simulink model "Demo_1_3Q_ST250"  (Simulink 7.7)
settings: Solver=ode4  StartTime=0.0  StopTime=inf  FixedStep=sample_time_Vicon  RelTol=1e-3
InitFcn:
  | sample_time_Vicon = 0.004;
  | sample_time=0.02;
  | DeltaT = sample_time;
  | H0 = -0.36;
  | Kl = 1;
  | Omega_r =1.1; %1.3
undefined symbols (not defined in the file or in its folder): DiscIntNeverNeededParam
libraries: simulink x19, dspadpt3 x8
(part 3 of 3)

== system Demo_1_3Q_ST250/Vicon_Data1/Raw Quad Pose from Vicon/Process Vicon Raw Data3/Flip_pi1/Flip_0_to_2pi ==
  Angle : Inport
  Add : Sum
  Compare To Constant1 : simulink/Logic and Bit Operations/Compare To Constant  SystemSampleTime=-1  relop=<  const=0  LogicOutDataTypeMode=uint8  ZeroCross=off
  Constant : Constant  Value=2*pi
  Data Type Duplicate : DataTypeDuplicate
  Flip_2pi : Subsystem
      mask Type: Flip -2pi to 2pi
      mask Description: Flips the inputs into the range -2pi to +2pi
      mask Help: Flips the inputs into the range -2pi to +2pi
      mask Display: disp('Flip_2pi')
  Switch : Switch  Criteria=u2 ~= 0
  Angle_Flip : Outport
  wires:
  Flip_2pi/1(Angle_Flip) -> Compare To Constant1/1, Add/2, Switch/3
  Compare To Constant1/1 -> Switch/2
  Constant/1 -> Add/1
  Add/1 -> Switch/1
  Angle/1 -> Flip_2pi/1(Angle), Data Type Duplicate/2
  Switch/1 -> Angle_Flip/1, Data Type Duplicate/1

== system Demo_1_3Q_ST250/Vicon_Data1/Raw Quad Pose from Vicon/Process Vicon Raw Data4/Flip_pi1/Flip_0_to_2pi ==
  Angle : Inport
  Add : Sum
  Compare To Constant1 : simulink/Logic and Bit Operations/Compare To Constant  SystemSampleTime=-1  relop=<  const=0  LogicOutDataTypeMode=uint8  ZeroCross=off
  Constant : Constant  Value=2*pi
  Data Type Duplicate : DataTypeDuplicate
  Flip_2pi : Subsystem
      mask Type: Flip -2pi to 2pi
      mask Description: Flips the inputs into the range -2pi to +2pi
      mask Help: Flips the inputs into the range -2pi to +2pi
      mask Display: disp('Flip_2pi')
  Switch : Switch  Criteria=u2 ~= 0
  Angle_Flip : Outport
  wires:
  Switch/1 -> Data Type Duplicate/1, Angle_Flip/1
  Angle/1 -> Data Type Duplicate/2, Flip_2pi/1(Angle)
  Add/1 -> Switch/1
  Constant/1 -> Add/1
  Compare To Constant1/1 -> Switch/2
  Flip_2pi/1(Angle_Flip) -> Switch/3, Add/2, Compare To Constant1/1

== system Demo_1_3Q_ST250/Vicon_Data1/Raw Quad Pose from Vicon/Process Vicon Raw Data5/Flip_pi1/Flip_0_to_2pi ==
  Angle : Inport
  Add : Sum
  Compare To Constant1 : simulink/Logic and Bit Operations/Compare To Constant  SystemSampleTime=-1  relop=<  const=0  LogicOutDataTypeMode=uint8  ZeroCross=off
  Constant : Constant  Value=2*pi
  Data Type Duplicate : DataTypeDuplicate
  Flip_2pi : Subsystem
      mask Type: Flip -2pi to 2pi
      mask Description: Flips the inputs into the range -2pi to +2pi
      mask Help: Flips the inputs into the range -2pi to +2pi
      mask Display: disp('Flip_2pi')
  Switch : Switch  Criteria=u2 ~= 0
  Angle_Flip : Outport
  wires:
  Switch/1 -> Data Type Duplicate/1, Angle_Flip/1
  Angle/1 -> Data Type Duplicate/2, Flip_2pi/1(Angle)
  Add/1 -> Switch/1
  Constant/1 -> Add/1
  Compare To Constant1/1 -> Switch/2
  Flip_2pi/1(Angle_Flip) -> Switch/3, Add/2, Compare To Constant1/1

== system Demo_1_3Q_ST250/Vicon_Data1/Raw Quad Pose from Vicon/Process Vicon Raw Data6/Flip_pi1/Flip_0_to_2pi ==
  Angle : Inport
  Add : Sum
  Compare To Constant1 : simulink/Logic and Bit Operations/Compare To Constant  SystemSampleTime=-1  relop=<  const=0  LogicOutDataTypeMode=uint8  ZeroCross=off
  Constant : Constant  Value=2*pi
  Data Type Duplicate : DataTypeDuplicate
  Flip_2pi : Subsystem
      mask Type: Flip -2pi to 2pi
      mask Description: Flips the inputs into the range -2pi to +2pi
      mask Help: Flips the inputs into the range -2pi to +2pi
      mask Display: disp('Flip_2pi')
  Switch : Switch  Criteria=u2 ~= 0
  Angle_Flip : Outport
  wires:
  Flip_2pi/1(Angle_Flip) -> Compare To Constant1/1, Add/2, Switch/3
  Compare To Constant1/1 -> Switch/2
  Constant/1 -> Add/1
  Add/1 -> Switch/1
  Angle/1 -> Flip_2pi/1(Angle), Data Type Duplicate/2
  Switch/1 -> Angle_Flip/1, Data Type Duplicate/1

== system Demo_1_3Q_ST250/Vicon_Data1/Raw Quad Pose from Vicon/Process Vicon Raw Data7/Flip_pi1/Flip_0_to_2pi ==
  Angle : Inport
  Add : Sum
  Compare To Constant1 : simulink/Logic and Bit Operations/Compare To Constant  SystemSampleTime=-1  relop=<  const=0  LogicOutDataTypeMode=uint8  ZeroCross=off
  Constant : Constant  Value=2*pi
  Data Type Duplicate : DataTypeDuplicate
  Flip_2pi : Subsystem
      mask Type: Flip -2pi to 2pi
      mask Description: Flips the inputs into the range -2pi to +2pi
      mask Help: Flips the inputs into the range -2pi to +2pi
      mask Display: disp('Flip_2pi')
  Switch : Switch  Criteria=u2 ~= 0
  Angle_Flip : Outport
  wires:
  Switch/1 -> Data Type Duplicate/1, Angle_Flip/1
  Angle/1 -> Data Type Duplicate/2, Flip_2pi/1(Angle)
  Add/1 -> Switch/1
  Constant/1 -> Add/1
  Compare To Constant1/1 -> Switch/2
  Flip_2pi/1(Angle_Flip) -> Switch/3, Add/2, Compare To Constant1/1

== system Demo_1_3Q_ST250/Vicon_Data1/Raw Quad Pose from Vicon/Process Vicon Raw Data8/Flip_pi1/Flip_0_to_2pi ==
  Angle : Inport
  Add : Sum
  Compare To Constant1 : simulink/Logic and Bit Operations/Compare To Constant  SystemSampleTime=-1  relop=<  const=0  LogicOutDataTypeMode=uint8  ZeroCross=off
  Constant : Constant  Value=2*pi
  Data Type Duplicate : DataTypeDuplicate
  Flip_2pi : Subsystem
      mask Type: Flip -2pi to 2pi
      mask Description: Flips the inputs into the range -2pi to +2pi
      mask Help: Flips the inputs into the range -2pi to +2pi
      mask Display: disp('Flip_2pi')
  Switch : Switch  Criteria=u2 ~= 0
  Angle_Flip : Outport
  wires:
  Flip_2pi/1(Angle_Flip) -> Compare To Constant1/1, Add/2, Switch/3
  Compare To Constant1/1 -> Switch/2
  Constant/1 -> Add/1
  Add/1 -> Switch/1
  Angle/1 -> Flip_2pi/1(Angle), Data Type Duplicate/2
  Switch/1 -> Angle_Flip/1, Data Type Duplicate/1

== system Demo_1_3Q_ST250/Vicon_Data1/Raw Quad Pose from Vicon/Process Vicon Raw Data1/Flip_pi1/Flip_0_to_2pi/Flip_2pi ==
  Angle : Inport
  Bias : Bias  Bias=-2*pi
  Constant : Constant  Value=2*pi
  Data Type Duplicate : DataTypeDuplicate
  Modulo : Math  Operator=mod  SaturateOnIntegerOverflow=on
  Sign1 : Signum
  Switch : Switch
  Angle_Flip : Outport
  wires:
  Angle/1 -> Modulo/1, Sign1/1, Data Type Duplicate/1
  Constant/1 -> Modulo/2
  Modulo/1 -> Bias/1, Switch/1
  Sign1/1 -> Switch/2
  Bias/1 -> Switch/3
  Switch/1 -> Angle_Flip/1, Data Type Duplicate/2

== system Demo_1_3Q_ST250/Vicon_Data1/Raw Quad Pose from Vicon/Process Vicon Raw Data2/Flip_pi1/Flip_0_to_2pi/Flip_2pi ==
  Angle : Inport
  Bias : Bias  Bias=-2*pi
  Constant : Constant  Value=2*pi
  Data Type Duplicate : DataTypeDuplicate
  Modulo : Math  Operator=mod  SaturateOnIntegerOverflow=on
  Sign1 : Signum
  Switch : Switch
  Angle_Flip : Outport
  wires:
  Switch/1 -> Data Type Duplicate/2, Angle_Flip/1
  Bias/1 -> Switch/3
  Sign1/1 -> Switch/2
  Modulo/1 -> Switch/1, Bias/1
  Constant/1 -> Modulo/2
  Angle/1 -> Data Type Duplicate/1, Sign1/1, Modulo/1

== system Demo_1_3Q_ST250/Vicon_Data1/Raw Quad Pose from Vicon/Process Vicon Raw Data3/Flip_pi1/Flip_0_to_2pi/Flip_2pi ==
  Angle : Inport
  Bias : Bias  Bias=-2*pi
  Constant : Constant  Value=2*pi
  Data Type Duplicate : DataTypeDuplicate
  Modulo : Math  Operator=mod  SaturateOnIntegerOverflow=on
  Sign1 : Signum
  Switch : Switch
  Angle_Flip : Outport
  wires:
  Angle/1 -> Modulo/1, Sign1/1, Data Type Duplicate/1
  Constant/1 -> Modulo/2
  Modulo/1 -> Bias/1, Switch/1
  Sign1/1 -> Switch/2
  Bias/1 -> Switch/3
  Switch/1 -> Angle_Flip/1, Data Type Duplicate/2

== system Demo_1_3Q_ST250/Vicon_Data1/Raw Quad Pose from Vicon/Process Vicon Raw Data4/Flip_pi1/Flip_0_to_2pi/Flip_2pi ==
  Angle : Inport
  Bias : Bias  Bias=-2*pi
  Constant : Constant  Value=2*pi
  Data Type Duplicate : DataTypeDuplicate
  Modulo : Math  Operator=mod  SaturateOnIntegerOverflow=on
  Sign1 : Signum
  Switch : Switch
  Angle_Flip : Outport
  wires:
  Switch/1 -> Data Type Duplicate/2, Angle_Flip/1
  Bias/1 -> Switch/3
  Sign1/1 -> Switch/2
  Modulo/1 -> Switch/1, Bias/1
  Constant/1 -> Modulo/2
  Angle/1 -> Data Type Duplicate/1, Sign1/1, Modulo/1

== system Demo_1_3Q_ST250/Vicon_Data1/Raw Quad Pose from Vicon/Process Vicon Raw Data5/Flip_pi1/Flip_0_to_2pi/Flip_2pi ==
  Angle : Inport
  Bias : Bias  Bias=-2*pi
  Constant : Constant  Value=2*pi
  Data Type Duplicate : DataTypeDuplicate
  Modulo : Math  Operator=mod  SaturateOnIntegerOverflow=on
  Sign1 : Signum
  Switch : Switch
  Angle_Flip : Outport
  wires:
  Switch/1 -> Data Type Duplicate/2, Angle_Flip/1
  Bias/1 -> Switch/3
  Sign1/1 -> Switch/2
  Modulo/1 -> Switch/1, Bias/1
  Constant/1 -> Modulo/2
  Angle/1 -> Data Type Duplicate/1, Sign1/1, Modulo/1

== system Demo_1_3Q_ST250/Vicon_Data1/Raw Quad Pose from Vicon/Process Vicon Raw Data6/Flip_pi1/Flip_0_to_2pi/Flip_2pi ==
  Angle : Inport
  Bias : Bias  Bias=-2*pi
  Constant : Constant  Value=2*pi
  Data Type Duplicate : DataTypeDuplicate
  Modulo : Math  Operator=mod  SaturateOnIntegerOverflow=on
  Sign1 : Signum
  Switch : Switch
  Angle_Flip : Outport
  wires:
  Angle/1 -> Modulo/1, Sign1/1, Data Type Duplicate/1
  Constant/1 -> Modulo/2
  Modulo/1 -> Bias/1, Switch/1
  Sign1/1 -> Switch/2
  Bias/1 -> Switch/3
  Switch/1 -> Angle_Flip/1, Data Type Duplicate/2

== system Demo_1_3Q_ST250/Vicon_Data1/Raw Quad Pose from Vicon/Process Vicon Raw Data7/Flip_pi1/Flip_0_to_2pi/Flip_2pi ==
  Angle : Inport
  Bias : Bias  Bias=-2*pi
  Constant : Constant  Value=2*pi
  Data Type Duplicate : DataTypeDuplicate
  Modulo : Math  Operator=mod  SaturateOnIntegerOverflow=on
  Sign1 : Signum
  Switch : Switch
  Angle_Flip : Outport
  wires:
  Switch/1 -> Data Type Duplicate/2, Angle_Flip/1
  Bias/1 -> Switch/3
  Sign1/1 -> Switch/2
  Modulo/1 -> Switch/1, Bias/1
  Constant/1 -> Modulo/2
  Angle/1 -> Data Type Duplicate/1, Sign1/1, Modulo/1

== system Demo_1_3Q_ST250/Vicon_Data1/Raw Quad Pose from Vicon/Process Vicon Raw Data8/Flip_pi1/Flip_0_to_2pi/Flip_2pi ==
  Angle : Inport
  Bias : Bias  Bias=-2*pi
  Constant : Constant  Value=2*pi
  Data Type Duplicate : DataTypeDuplicate
  Modulo : Math  Operator=mod  SaturateOnIntegerOverflow=on
  Sign1 : Signum
  Switch : Switch
  Angle_Flip : Outport
  wires:
  Angle/1 -> Modulo/1, Sign1/1, Data Type Duplicate/1
  Constant/1 -> Modulo/2
  Modulo/1 -> Bias/1, Switch/1
  Sign1/1 -> Switch/2
  Bias/1 -> Switch/3
  Switch/1 -> Angle_Flip/1, Data Type Duplicate/2

== matlab function Quad 1 Planning/Yaw Controller/MATLAB Function ==
  data: u input double; y output double
function y = fcn(u)
%#codegen
y = u;
if y > pi    
    y = y - 2*pi;
elseif y < -pi
        y = y + 2*pi;
end

== stateflow chart Quad 2 Planning/Trajectory Logic/UAV SF ==
  state Landing
    state Decsending
      en:PosDesired = Pos;
      du:PosDesired[2] = (0 - PosDesired[2])*1*DeltaT + PosDesired[2] ;
    state CutThrottle
      du:HoverThrottle = (-0.95 - HoverThrottle)*2*DeltaT + HoverThrottle ;
    (default) -> Decsending
    Decsending -> CutThrottle : [Pos[2] > -0.15]
  state Airborne
    state TakeOff
      du:HoverThrottle = (H0 - HoverThrottle)*2*DeltaT + HoverThrottle ;
    state Hover
      en: PosDesired[2] = -1;
    state Line
      state Waypoint2
        en: PosDesired[0] = 0; PosDesired[1] = -1.7321-0.5;  PosDesired[2] = -2;
      state Waypoint1
        en: PosDesired[0] = 0; PosDesired[1] = 1.7321-0.5; PosDesired[2] = -1;
        line_count = line_count+1;
      (default) -> Airborne.Line.Waypoint1 : {line_count = -1;}
      Airborne.Line.Waypoint2 -> Airborne.Line.Waypoint1 : after(5,sec)
      Airborne.Line.Waypoint1 -> Airborne.Line.Waypoint2 : after(5,sec)
    state Triangle_CW
      state Waypoint3
        en:PosDesired[0] = -2;
        PosDesired[1] = 1.7321-0.5;
        PosDesired[2] = -1;
      state Waypoint2
        en:PosDesired[0] = 2;
        PosDesired[1] = 1.7321-0.5;
        PosDesired[2] = -1.5;
        triangle_count = triangle_count + 1;
      state Waypoint1
        en:PosDesired[0] = 0;
        PosDesired[1] = -1.7321-0.5;
        PosDesired[2] = -2.0;
      (default) -> Airborne.Triangle_CW.Waypoint2 : {triangle_count = -1;}
      Airborne.Triangle_CW.Waypoint3 -> Airborne.Triangle_CW.Waypoint1 : after(5,sec)
      Airborne.Triangle_CW.Waypoint2 -> Airborne.Triangle_CW.Waypoint3 : after(5,sec)
      Airborne.Triangle_CW.Waypoint1 -> Airborne.Triangle_CW.Waypoint2 : after(5,sec)
    state Triangle_CCW
      state Waypoint3
        en:PosDesired[0] = 2;
        PosDesired[1] = 1.7321-0.5;
        PosDesired[2] = -1.5;
      state Waypoint1
        en:PosDesired[0] = 0;
        PosDesired[1] = -1.7321-0.5;
        PosDesired[2] = -2.0;
      state Waypoint2
        en:PosDesired[0] = -2;
        PosDesired[1] = 1.7321-0.5;
        PosDesired[2] = -1;
        triangle_count = triangle_count + 1;
      Airborne.Triangle_CCW.Waypoint3 -> Airborne.Triangle_CCW.Waypoint1 : after(5,sec)
      (default) -> Airborne.Triangle_CCW.Waypoint1 : {triangle_count = -1;}
      Airborne.Triangle_CCW.Waypoint2 -> Airborne.Triangle_CCW.Waypoint3 : after(5,sec)
      Airborne.Triangle_CCW.Waypoint1 -> Airborne.Triangle_CCW.Waypoint2 : after(5,sec)
    (default) -> TakeOff : {PosDesired = Pos;  PosDesired[2] = -1;}
    TakeOff -> Hover : after(5,sec)
        | {PosDesired = Pos;}
    Hover -> Line : [RC[5] > 0]
    Triangle_CW -> Hover [order 2] : [RC[5] < 0]
        | {PosDesired = Pos;}
    Line -> Triangle_CCW [order 1] : [line_count == 2]
    Line -> Hover [order 2] : [RC[5] < 0]
        | {PosDesired = Pos;}
    Triangle_CW -> Hover [order 1] : [triangle_count == 2]
    Triangle_CCW -> Hover [order 1] : [RC[5] < 0]
        | {PosDesired = Pos;}
    Triangle_CCW -> Triangle_CW [order 2] : [triangle_count == 2]
  (default) -> Landing : {HoverThrottle=-0.95;}
  Airborne -> Landing : [RC[6] < -0.5]
  Landing -> Airborne : [RC[6] > 0.5]
  data: PosDesired output double size=4; HoverThrottle output double size=1; Mode output uint8 size=3; RC input double size=8; Pos input double size=4; PerchPos input double size=4; DeltaT parameter double size=1; H0 parameter double size=1; Kl parameter double size=1; VelCmd local double size=2 =0; line_count local int8 size=1 =0; triangle_count local int8 size=1 =0

== stateflow chart Quad 1 Planning/Trajectory Logic/UAV SF ==
  state Landing
    state Decsending
      en:PosDesired = Pos;
      du:PosDesired[2] = (0 - PosDesired[2])*1*DeltaT + PosDesired[2] ;
    state CutThrottle
      du:HoverThrottle = (-0.95 - HoverThrottle)*2*DeltaT + HoverThrottle ;
    (default) -> Decsending
    Decsending -> CutThrottle : [Pos[2] > -0.15]
  state Airborne
    state TakeOff
      du:HoverThrottle = (H0 - HoverThrottle)*2*DeltaT + HoverThrottle ;
    state Hover
      en: PosDesired[2] = -1;
    state Line
      state Waypoint2
        en: PosDesired[0] = 2; PosDesired[1] = -1.7321-0.5;  PosDesired[2] = -2;
      state Waypoint1
        en: PosDesired[0] = 2; PosDesired[1] = 1.7321-0.5; PosDesired[2] = -1;
        line_count = line_count+1;
      (default) -> Airborne.Line.Waypoint1 : {line_count = -1;}
      Airborne.Line.Waypoint2 -> Airborne.Line.Waypoint1 : after(5,sec)
      Airborne.Line.Waypoint1 -> Airborne.Line.Waypoint2 : after(5,sec)
    state Triangle_CW
      state Waypoint2
        en:PosDesired[0] = -2;
        PosDesired[1] = 1.7321-0.5;
        PosDesired[2] = -1;
        triangle_count = triangle_count + 1;
      state Waypoint1
        en:PosDesired[0] = 2;
        PosDesired[1] = 1.7321-0.5;
        PosDesired[2] = -1.5;
      state Waypoint3
        en:PosDesired[0] = 0;
        PosDesired[1] = -1.7321-0.5;
        PosDesired[2] = -2.0;
      (default) -> Airborne.Triangle_CW.Waypoint2 : {triangle_count = -1;}
      Airborne.Triangle_CW.Waypoint1 -> Airborne.Triangle_CW.Waypoint2 : after(5,sec)
      Airborne.Triangle_CW.Waypoint2 -> Airborne.Triangle_CW.Waypoint3 : after(5,sec)
      Airborne.Triangle_CW.Waypoint3 -> Airborne.Triangle_CW.Waypoint1 : after(5,sec)
    state Triangle_CCW
      state Waypoint3
        en:PosDesired[0] = -2;
        PosDesired[1] = 1.7321-0.5;
        PosDesired[2] = -1;
      state Waypoint1
        en:PosDesired[0] = 2;
        PosDesired[1] = 1.7321-0.5;
        PosDesired[2] = -1.5;
      state Waypoint2
        en:PosDesired[0] = 0;
        PosDesired[1] = -1.7321-0.5;
        PosDesired[2] = -2.0;
        triangle_count = triangle_count + 1;
      Airborne.Triangle_CCW.Waypoint1 -> Airborne.Triangle_CCW.Waypoint2 : after(5,sec)
      Airborne.Triangle_CCW.Waypoint3 -> Airborne.Triangle_CCW.Waypoint1 : after(5,sec)
      (default) -> Airborne.Triangle_CCW.Waypoint1 : {triangle_count = -1;}
      Airborne.Triangle_CCW.Waypoint2 -> Airborne.Triangle_CCW.Waypoint3 : after(5,sec)
    (default) -> TakeOff : {PosDesired = Pos;  PosDesired[2] = -1;}
    TakeOff -> Hover : after(5,sec)
        | {PosDesired = Pos;}
    Hover -> Line : [RC[5] > 0]
    Triangle_CW -> Hover [order 2] : [RC[5] < 0]
        | {PosDesired = Pos;}
    Triangle_CCW -> Triangle_CW [order 2] : [triangle_count == 2]
    Triangle_CCW -> Hover [order 1] : [RC[5] < 0]
        | {PosDesired = Pos;}
    Line -> Triangle_CCW [order 1] : [line_count == 2]
    Line -> Hover [order 2] : [RC[5] < 0]
        | {PosDesired = Pos;}
    Triangle_CW -> Hover [order 1] : [triangle_count == 2]
  (default) -> Landing : {HoverThrottle=-0.95;}
  Airborne -> Landing : [RC[6] < -0.5]
  Landing -> Airborne : [RC[6] > 0.5]
  data: PosDesired output double size=4; HoverThrottle output double size=1; Mode output uint8 size=3; RC input double size=8; Pos input double size=4; PerchPos input double size=4; DeltaT parameter double size=1; H0 parameter double size=1; Kl parameter double size=1; VelCmd local double size=2 =0; line_count local int8 size=1 =0; triangle_count local int8 size=1 =0

== matlab function Quad 2 Planning/Yaw Controller/MATLAB Function ==
  data: u input double; y output double
function y = fcn(u)
%#codegen
y = u;
if y > pi    
    y = y - 2*pi;
elseif y < -pi
        y = y + 2*pi;
end

== stateflow chart Quad 4 Planning (same as Q3)/Trajectory Logic/UAV SF ==
  state Landing
    state Decsending
      en:PosDesired = Pos;
      du:PosDesired[2] = (0 - PosDesired[2])*1*DeltaT + PosDesired[2] ;
    state CutThrottle
      du:HoverThrottle = (-0.95 - HoverThrottle)*2*DeltaT + HoverThrottle ;
    (default) -> Decsending
    Decsending -> CutThrottle : [Pos[2] > -0.15]
  state Airborne
    state TakeOff
      du:HoverThrottle = (-0.27 - HoverThrottle)*2*DeltaT + HoverThrottle ;
    state Hover
      en: PosDesired[2] = -1;
    state Line
      state Waypoint2
        en: PosDesired[0] = -2; PosDesired[1] = -1.7321-0.5;  PosDesired[2] = -2;
      state Waypoint1
        en: PosDesired[0] = -2; PosDesired[1] = 1.7321-0.5; PosDesired[2] = -1;
        line_count = line_count+1;
      (default) -> Airborne.Line.Waypoint1 : {line_count = -1;}
      Airborne.Line.Waypoint2 -> Airborne.Line.Waypoint1 : after(5,sec)
      Airborne.Line.Waypoint1 -> Airborne.Line.Waypoint2 : after(5,sec)
    state Triangle_CW
      state Waypoint3
        en:PosDesired[0] = 2;
        PosDesired[1] = 1.7321-0.5;
        PosDesired[2] = -1.5;
      state Waypoint2
        en:PosDesired[0] = 0;
        PosDesired[1] = -1.7321-0.5;
        PosDesired[2] = -2.0;
        triangle_count = triangle_count + 1;
      state Waypoint1
        en:PosDesired[0] = -2;
        PosDesired[1] = 1.7321-0.5;
        PosDesired[2] = -1;
      (default) -> Airborne.Triangle_CW.Waypoint2 : {triangle_count = -1;}
      Airborne.Triangle_CW.Waypoint3 -> Airborne.Triangle_CW.Waypoint1 : after(5,sec)
      Airborne.Triangle_CW.Waypoint2 -> Airborne.Triangle_CW.Waypoint3 : after(5,sec)
      Airborne.Triangle_CW.Waypoint1 -> Airborne.Triangle_CW.Waypoint2 : after(5,sec)
    state Triangle_CCW
      state Waypoint3
        en:PosDesired[0] = 0;
        PosDesired[1] = -1.7321-0.5;
        PosDesired[2] = -2.0;
      state Waypoint1
        en:PosDesired[0] = -2;
        PosDesired[1] = 1.7321-0.5;
        PosDesired[2] = -1;
      state Waypoint2
        en:PosDesired[0] = 2;
        PosDesired[1] = 1.7321-0.5;
        PosDesired[2] = -1.5;
        triangle_count = triangle_count + 1;
      Airborne.Triangle_CCW.Waypoint3 -> Airborne.Triangle_CCW.Waypoint1 : after(5,sec)
      (default) -> Airborne.Triangle_CCW.Waypoint1 : {triangle_count = -1;}
      Airborne.Triangle_CCW.Waypoint2 -> Airborne.Triangle_CCW.Waypoint3 : after(5,sec)
      Airborne.Triangle_CCW.Waypoint1 -> Airborne.Triangle_CCW.Waypoint2 : after(5,sec)
    (default) -> TakeOff : {PosDesired = Pos;  PosDesired[2] = -1;}
    TakeOff -> Hover : after(5,sec)
        | {PosDesired = Pos;}
    Hover -> Line : [RC[5] > 0]
    Triangle_CW -> Hover [order 2] : [RC[5] < 0]
        | {PosDesired = Pos;}
    Line -> Triangle_CCW [order 1] : [line_count == 2]
    Line -> Hover [order 2] : [RC[5] < 0]
        | {PosDesired = Pos;}
    Triangle_CW -> Hover [order 1] : [triangle_count == 2]
    Triangle_CCW -> Hover [order 1] : [RC[5] < 0]
        | {PosDesired = Pos;}
    Triangle_CCW -> Triangle_CW [order 2] : [triangle_count == 2]
  (default) -> Landing : {HoverThrottle=-0.95;}
  Airborne -> Landing : [RC[6] < -0.5]
  Landing -> Airborne : [RC[6] > 0.5]
  data: PosDesired output double size=4; HoverThrottle output double size=1; Mode output uint8 size=3; RC input double size=8; Pos input double size=4; PerchPos input double size=4; DeltaT parameter double size=1; H0 parameter double size=1; Kl parameter double size=1; VelCmd local double size=2 =0; line_count local int8 size=1 =0; triangle_count local int8 size=1 =0

== matlab function Quad 4 Planning (same as Q3)/Yaw Controller/MATLAB Function ==
  data: u input double; y output double
function y = fcn(u)
%#codegen
y = u;
if y > pi    
    y = y - 2*pi;
elseif y < -pi
        y = y + 2*pi;
end
